simulink library "uavsimBlockset_StateSpaceSystem"  (Simulink 8.0)
settings: Solver=ode45  StartTime=0.0  StopTime=10.0  RelTol=1e-3
settings Model: Creator=mstolle  LastModifiedBy=j.bolting

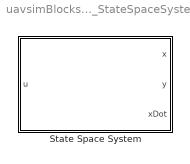
== system uavsimBlockset_StateSpaceSystem ==
  State Space System : Subsystem  mask{mask_a=0, mask_b=0, mask_c=0, mask_d=0, mask_x0=0}
      mask prompts: mask_a "Dynamic matrix A"; mask_b "Input matrix B"; mask_c "Output matrix C"; mask_d "Feedthrough matrix D"; mask_x0 "Initial state x0"

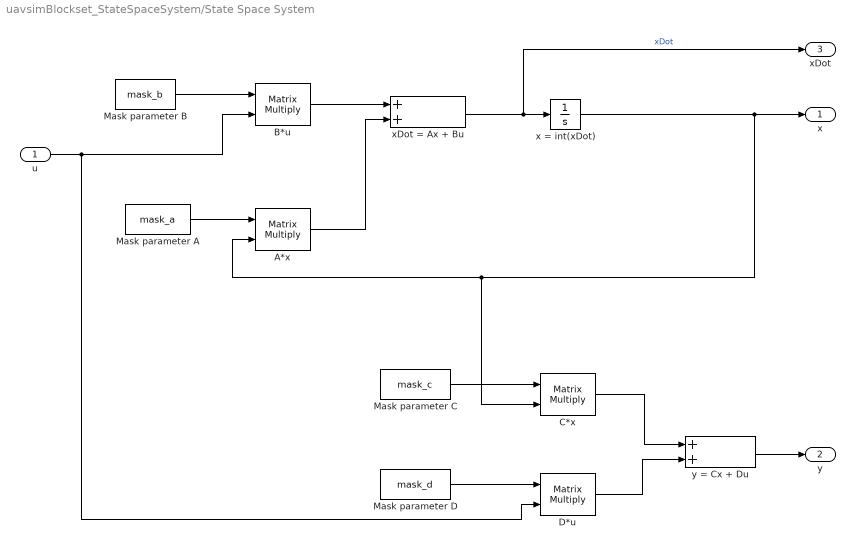
== system uavsimBlockset_StateSpaceSystem/State Space System ==
  u : Inport
  A*x : Product  Multiplication=Matrix(*)
  B*u : Product  Multiplication=Matrix(*)
  C*x : Product  Multiplication=Matrix(*)
  D*u : Product  Multiplication=Matrix(*)
  Mask parameter A : Constant  Value=mask_a
  Mask parameter B : Constant  Value=mask_b
  Mask parameter C : Constant  Value=mask_c
  Mask parameter D : Constant  Value=mask_d
  x = int(xDot) : Integrator  InitialCondition=mask_x0
  xDot = Ax + Bu : Sum
  y = Cx + Du : Sum
  x : Outport
  y : Outport  Port=2
  xDot : Outport  Port=3
  wires:
  Mask parameter B/1 -> B*u/1
  u/1 -> B*u/2, D*u/2
  B*u/1 -> xDot = Ax + Bu/1
  xDot = Ax + Bu/1 -> xDot/1, x = int(xDot)/1  "xDot"
  Mask parameter A/1 -> A*x/1
  A*x/1 -> xDot = Ax + Bu/2
  Mask parameter D/1 -> D*u/1
  C*x/1 -> y = Cx + Du/1
  D*u/1 -> y = Cx + Du/2
  y = Cx + Du/1 -> y/1
  x = int(xDot)/1 -> x/1, C*x/2, A*x/2
  Mask parameter C/1 -> C*x/1
